simulink model "Kubon_lab10_sim"  (R2020b)
settings: Solver=VariableStepAuto  StartTime=0.0  StopTime=T_stop  RelTol=1e-3
values from neighbouring files (symbols this model uses):
  cpN = 1000    [Kubon_lab10.m]    (also in Kubon_lab13.m; Kubon_lab9.m; mini_v1.m)
  Cv1 = cpN*ppN*V1N    (= 21000)    [Kubon_lab10.m]    (also in Kubon_lab13.m; Kubon_lab9.m)
  Cv2 = cpN*ppN*V2N    (= 14700)    [Kubon_lab10.m]    (also in Kubon_lab13.m; Kubon_lab9.m)
  dfkz = 0.0    (= 0)    [Kubon_lab10.m]    (also in Kubon_lab9.m)
  dTkz = 2.0    (= 2)    [Kubon_lab10.m]    (also in Kubon_lab9.m = 0)
  dTzew = 0.0    (= 0)    [Kubon_lab10.m]    (also in Kubon_lab9.m)
  fk0 = fkN *0.7    (= 0.7)    [Kubon_lab10.m]    (also in Kubon_lab13.m = 1; Kubon_lab9.m = 1)
  k0 = ((cpN*ppN*fkN)*(TkzN-Tw1N)-ks1*(Tw1N-TzewN))/(Tw1N-Tw2N)    (= 480)    [Kubon_lab10.m]    (also in Kubon_lab13.m; Kubon_lab9.m)
  ks1 = (cpN*ppN*fkN*(TkzN-Tw2N))/(Tw1N-2*TzewN+Tw2N)    (= 240)    [Kubon_lab10.m]    (also in Kubon_lab13.m; Kubon_lab9.m)
  ks2 = ks1    (= 240)    [Kubon_lab10.m]    (also in Kubon_lab13.m; Kubon_lab9.m)
  ppN = 1.2    [Kubon_lab10.m]    (also in Kubon_lab13.m; Kubon_lab9.m; mini_v1.m)
  t0 = 50.0    (= 50)    [Kubon_lab10.m]    (also in Kubon_lab4.m = 5; Kubon_lab5.m = 0; Kubon_lab6.m = 5; Kubon_lab6_test.m = 0)
  Tkz0 = TkzN*0.7    (= 21)    [Kubon_lab10.m]    (also in Kubon_lab9.m = 30)
  Tw10 = ( (a_1*b_1*Tkz0)+ks1*(ks1+a_1+2*k0)*Tzew0 )/( (b_1^2)-(k0*(k0+a_1)) )    (= 9.848)    [Kubon_lab10.m]    (also in Kubon_lab9.m = 20)
  Tw20 = ( (k0+a_1)*Tw10+ks1*Tzew0 )/( k0+a_1+ks1 )    (= 5.256)    [Kubon_lab10.m]    (also in Kubon_lab9.m = 15)
  Tzew0 = TzewN    (= -20)    [Kubon_lab10.m]    (also in Kubon_lab9.m)
settings Model: Creator=pkubo  LastModifiedBy=pkubo

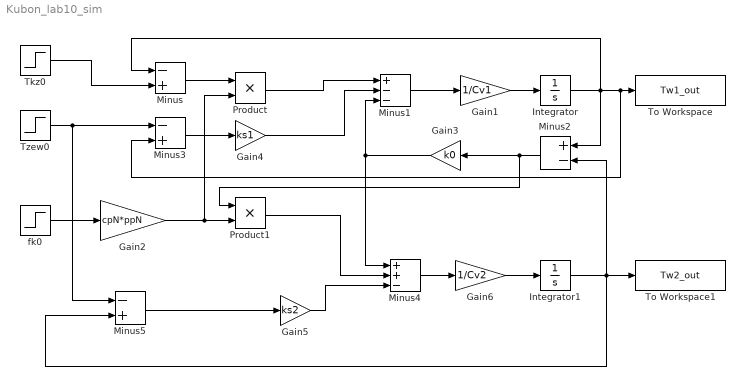
== system Kubon_lab10_sim ==
  Gain1 : Gain  Gain=1/Cv1
  Gain2 : Gain  Gain=cpN*ppN
  Gain3 : Gain  Gain=k0
  Gain4 : Gain  Gain=ks1
  Gain5 : Gain  Gain=ks2
  Gain6 : Gain  Gain=1/Cv2
  Integrator : Integrator  InitialCondition=Tw10
  Integrator1 : Integrator  InitialCondition=Tw20
  Minus : Sum  Inputs=-+
  Minus1 : Sum  Inputs=+--
  Minus2 : Sum  Inputs=+-
  Minus3 : Sum  Inputs=-+
  Minus4 : Sum  Inputs=++-
  Minus5 : Sum  Inputs=-+
  Product : Product
  Product1 : Product
  Tkz0 : Step  Time=t0  Before=Tkz0  After=Tkz0+dTkz  SampleTime=0
  To Workspace : ToWorkspace  VariableName=Tw1_out  SampleTime=-1
  To Workspace1 : ToWorkspace  VariableName=Tw2_out  SampleTime=-1
  Tzew0 : Step  Time=t0  Before=Tzew0  After=Tzew0+dTzew  SampleTime=0
  fk0 : Step  Time=t0  Before=fk0  After=fk0+dfkz  SampleTime=0
  wires:
  Minus/1 -> Product/1
  Minus1/1 -> Gain1/1
  Gain1/1 -> Integrator/1
  Integrator/1 -> Minus/1, Minus2/1, Minus3/2, To Workspace/1
  Product/1 -> Minus1/1
  fk0/1 -> Gain2/1
  Gain2/1 -> Product1/2, Product/2
  Minus3/1 -> Gain4/1
  Gain4/1 -> Minus1/2
  Minus2/1 -> Product1/1, Gain3/1
  Tkz0/1 -> Minus/2
  Tzew0/1 -> Minus5/1, Minus3/1
  Minus5/1 -> Gain5/1
  Gain5/1 -> Minus4/3
  Minus4/1 -> Gain6/1
  Gain6/1 -> Integrator1/1
  Integrator1/1 -> Minus2/2, Minus5/2, To Workspace1/1
  Gain3/1 -> Minus4/1, Minus1/3
  Product1/1 -> Minus4/2
